simulink model "blinky"  (R2025a)
settings: Solver=FixedStepDiscrete  StartTime=0.0  StopTime=inf  FixedStep=0.001  RelTol=1e-3
model workspace (MAT data in the model file):
  active = Simulink.Parameter
  active.Value = 1
  active.Complexity = 'real'
  active.Dimensions = [1 1]
  active.DataType = 'uint8'
  inactive = Simulink.Parameter
  inactive.Value = 0
  inactive.Complexity = 'real'
  inactive.Dimensions = [1 1]
  inactive.DataType = 'uint8'
undefined symbols (not defined in the file or in its folder): CR, LF, PWM_MAX, PWM_MIN, SPEED_Kd, SPEED_Ki, SPEED_Kp
libraries: instrumentseriallib x3, slpidlib x2, simulink x1, SignalEditorBlockLib x1
settings Model: DataDictionary=control_motor.sldd  Creator=g'w'c  LastModifiedBy=g'w'c
settings OptimizationCC: DefaultParameterBehavior=Inlined  UseDivisionForNetSlopeComputation=on  GainParamInheritBuiltInType=on  UseFloatMulNetSlope=on  DefaultUnderspecifiedDataType=single  InlineInvariantSignals=on  PassReuseOutputArgsAs=Individual arguments  ActiveStateOutputEnumStorageType=uint8  ZeroExternalMemoryAtStartup=off  ZeroInternalMemoryAtStartup=off  NoFixptDivByZeroProtection=on  EfficientFloat2IntCast=on  LifeSpan=1  OptimizeBlockOrder=speed  DifferentSizesBufferReuse=on  EfficientTunableParamExpr=on
settings DebuggingCC: ParameterTunabilityLossMsg=error
settings HardwareCC: ProdLongLongMode=on
settings SFSimCC: MATLABDynamicMemAlloc=off
settings RTWCC: SystemTargetFile=ert.tlc  GenCodeOnly=on  TemplateMakefile=ert_default_tmf  GenerateReport=on  IncludeHyperlinkInReport=on  LaunchReport=on  GenerateTraceInfo=on  GenerateCodeMetricsReport=on  Description=Embedded Coder
settings CodeAppCC: ForceParamTrailComments=on  IgnoreCustomStorageClasses=off  OperatorAnnotations=on  SimulinkDataObjDesc=on  SFDataObjDesc=on  CustomSymbolStrGlobalVar=rt$N$M  CustomSymbolStrType=$N$M  CustomSymbolStrFcn=$N$M$F  CustomSymbolStrMacro=$N$M  InsertBlockDesc=on
settings ERTTargetCC: ExtModeTransport=0.0  ExtModeStaticAlloc=off  ExtModeMexFile=ext_comm  ExtModeIntrfLevel=Level1  ERTCustomFileTemplate=example_file_process.tlc  ERTFilePackagingFormat=CompactWithDataFile  TargetLangStandard=C99 (ISO)  GenerateSampleERTMain=on  IncludeMdlTerminateFcn=off  CombineSignalStateStructs=on  PurelyIntegerCode=on  SupportNonFinite=off  SupportComplex=off  SupportNonInlinedSFcns=on

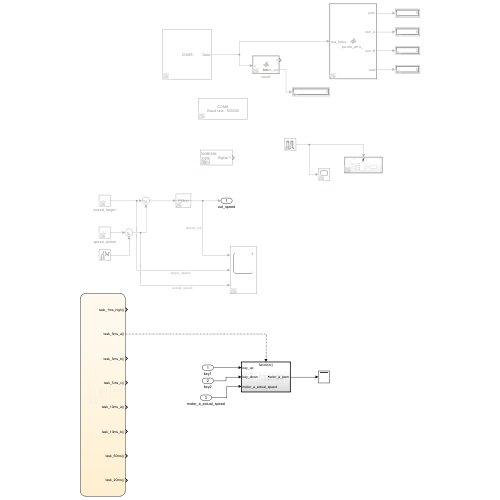
[thumbnail: Simulink's stored preview of the top-level diagram]
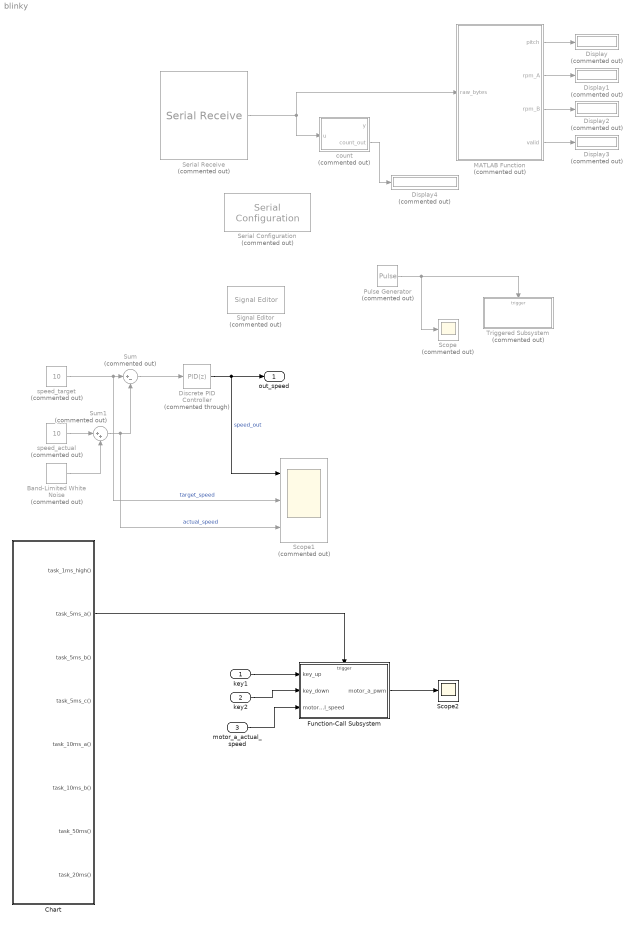
== system blinky ==
  key1 : Inport
  key2 : Inport  Port=2
  motor_a_actual_speed : Inport  Port=3
  Band-Limited White Noise : simulink/Sources/Band-Limited White Noise  Commented=on  Cov=[0.1]  Ts=0.1  seed=[23341]
  Chart : Stateflow chart  TreatAsAtomicUnit=on
  Discrete PID Controller : slpidlib/PID Controller  Commented=through  Controller=PID  Form=Parallel  TimeDomain=Discrete-time  UseExternalTs=off  SampleTime=-1  IntegratorMethod=Forward Euler  FilterMethod=Forward Euler  ControllerParametersSource=internal  P=1  I=1  UseKiTs=off  D=0  UseExternalDerivativeSource=off  N=100  UseFilter=on  TunerSelectOption=Transfer Function Based (PID Tuner App)  InitialConditionSource=internal  InitialConditionForIntegrator=0  InitialConditionForFilter=0  DifferentiatorICPrevScaledInput=0  ExternalReset=none  TrackingMode=off  Kt=1  LimitOutput=off  SatLimitsSource=internal  UpperSaturationLimit=inf  LowerSaturationLimit=-inf  LinearizeAsGain=off  AntiWindupMode=none  Kb=1  LimitIntegrator=off  UpperIntegratorSaturationLimit=inf  LowerIntegratorSaturationLimit=-inf  POutMin=[]  POutMax=[]  IOutMin=[]  IOutMax=[]  DOutMin=[]  DOutMax=[]  NOutMin=[]  NOutMax=[]  SumOutMin=[]  SumOutMax=[]  SaturationOutMin=[]  SaturationOutMax=[]  PParamMin=[]  PParamMax=[]  IParamMin=[]  IParamMax=[]  DParamMin=[]  DParamMax=[]  NParamMin=[]  NParamMax=[]  KbParamMin=[]  KbParamMax=[]  KtParamMin=[]  KtParamMax=[]  KbOutMin=[]  KbOutMax=[]  KtOutMin=[]  KtOutMax=[]  IntegratorOutMin=[]  IntegratorOutMax=[]  FilterOutMin=[]  FilterOutMax=[]  SumI1OutMin=[]  SumI1OutMax=[]  SumI2OutMin=[]  SumI2OutMax=[]  SumI3OutMin=[]  SumI3OutMax=[]  SumI4OutMin=[]  SumI4OutMax=[]  SumDOutMin=[]  SumDOutMax=[]  DifferentiatorOutMin=[]  DifferentiatorOutMax=[]  FilterDiffOutCoefMin=[]  FilterDiffOutCoefMax=[]  ReciprocalOutMin=[]  ReciprocalOutMax=[]  SumDenOutMin=[]  SumDenOutMax=[]  SumNumOutMin=[]  SumNumOutMax=[]  DivideOutMin=[]  DivideOutMax=[]  UdiffTsProdOutMin=[]  UdiffTsProdOutMax=[]  NTsProdOutMin=[]  NTsProdOutMax=[]  UintegralTsProdOutMin=[]  UintegralTsProdOutMax=[]  UngainTsProdOutMin=[]  UngainTsProdOutMax=[]  ClampingZeroOutDataTypeStr=Inherit: Inherit via back propagation  ClampingZeroOutMin=[]  ClampingZeroOutMax=[]  FilterDenConstantOutDataTypeStr=Inherit: Inherit via back propagation  FilterDenConstantOutMin=[]  FilterDenConstantOutMax=[]  PCopyOutDataTypeStr=Inherit: Inherit via back propagation  PCopyOutMin=[]  PCopyOutMax=[]  NCopyOutDataTypeStr=Inherit: Inherit via back propagation  NCopyOutMin=[]  NCopyOutMax=[]  IntegratorContinuousStateAttributes=''  IntegratorStateMustResolveToSignalObject=off  IntegratorRTWStateStorageClass=Auto  FilterContinuousStateAttributes=''  FilterStateMustResolveToSignalObject=off  FilterRTWStateStorageClass=Auto  ParallelPVariant=InternalParameters  IdealPVariant=Disabled  IVariant=InternalParameters  DVariant=InternalParameters  IntegratorVariant=Discrete  SatVariant=Disabled  AWVariant=Passthrough  PCopyVariant=Disabled  TRVariant=Disabled  FdbkBlocksVariant=Forward  IdealPFdbkVariant=Disabled  SatFdbkVariant=Disabled  DerivativeFilterVariant=ForwardEulerFilter  NVariant=InternalParameters  NCopyVariant=Disabled  FilterICVariant=InternalICsFilter  IntegratorICVariant=InternalICs  ExternalResetVariant=Disabled  TRSumVariant=Passthrough  SumFdbkVariant=Disabled  SumVariant=Sum_PID  TsampFilterVariant=InternalTs  TsampNgainVariant=Passthrough  TsampIntegralVariant=Disabled_SignalSpec  ExternalSaturationOutDataTypeStr=Inherit: Same as second input  DerivativeSourceVariant=ErrorSignal  PreIntVariant=InternalPreInt
      settings: LibrarySourceBlock=simulink/Discrete/Discrete PID Controller
  Display{,1..4} (5 alike) : Display  Commented=on
      Display4 settings: Format=decimal (Stored Integer)
  Function-Call Subsystem : Subsystem  TreatAsAtomicUnit=on
  MATLAB Function : MATLAB Function  Commented=on  TreatAsAtomicUnit=on
  Pulse Generator : DiscretePulseGenerator  Commented=on  PulseType=Time based  Period=1
  Scope : Scope  Commented=on
      settings: ActiveDisplayYMinimum=-4.2942185236028347  ActiveDisplayYMaximum=2.5004399483972364
  Scope1 : Scope  Commented=on  NumInputPorts=3
      settings: ActiveDisplayYMinimum=-1.2558823787460671E+274  ActiveDisplayYMaximum=2.7568149777352689E+273
  Scope2 : Scope
      settings: DataLoggingVariableName=ScopeData3
  Serial Configuration : instrumentseriallib/Serial Configuration  Priority=-200000  Commented=on  PortSel=COM8  Port=COM8  ComPort=COM8  BaudRate=500000  DataBits=8  Parity=none  StopBits=1  ByteOrder=little-endian  FlowControl=none  Timeout=10  SimulateUsing=Interpreted execution  BlockInModel=on  aMode=1
  Serial Receive : instrumentseriallib/Serial Receive  Priority=1  Commented=on  PortSel=COM8  Port=COM8  ComPort=COM8  DataType=uint8  SaveDataType=uint8  ToggleHeader=on  Header=[170 255]  ToggleDataSize=on  DataSize=[1 30]  ToggleTerminator=off  Terminator=CR/LF ('\r\n')  CustomTerminator=[]  InputFormat=Column major  EnableBlockingMode=on  ActionDataUnavailable=Output last received value  ActionWhenDataUnavailable=Output last received value  CustomValue=0  SampleTime=0.01  SimulateUsing=Interpreted execution  BlockInModel=on  aMode=1  LibraryInUse=instrumentlib
  Signal Editor : SignalEditorBlockLib/Signal Editor  Commented=on  FileName=com_uart.mat  ActiveScenario=Scenario  ActiveSignal=Signal 1  IsBus=off  OutputBusObjectStr=Bus: BusObject  SampleTime=0  ZeroCross=off  OutputAfterFinalValue=Setting to zero  Unit=inherit  PreserveSignalName=on  ApplySigPropsToAllScenarios=on  ApplySigPropsToAllSignals=off  SignalPropertySource=Dialog parameters
  Sum : Sum  Commented=on  Inputs=|+-
  Sum1 : Sum  Commented=on  Inputs=|++
  Triggered Subsystem : Subsystem  Commented=on  TreatAsAtomicUnit=on
  count : MATLAB Function  Commented=on  TreatAsAtomicUnit=on
  speed_actual : Constant  Commented=on  Value=10
  speed_target : Constant  Commented=on  Value=10
  out_speed : Outport
  wires:
  Serial Receive/1 -> MATLAB Function/1(raw_bytes), count/1(u)
  Pulse Generator/1 -> Triggered Subsystem/Trigger, Scope/1
  count/2(count_out) -> Display4/1
  MATLAB Function/1(pitch) -> Display/1
  MATLAB Function/2(rpm_A) -> Display1/1
  MATLAB Function/3(rpm_B) -> Display2/1
  MATLAB Function/4(valid) -> Display3/1
  speed_target/1 -> Scope1/2, Sum/1  "target_speed"
  Sum/1 -> Discrete PID Controller/1
  speed_actual/1 -> Sum1/1
  Band-Limited White Noise/1 -> Sum1/2
  Sum1/1 -> Scope1/3, Sum/2  "actual_speed"
  Discrete PID Controller/1 -> Scope1/1, out_speed/1  "speed_out"
  Chart/2(task_5ms_a()) -> Function-Call Subsystem/Trigger
  key1/1 -> Function-Call Subsystem/1(key_up)
  key2/1 -> Function-Call Subsystem/2(key_down)
  motor_a_actual_speed/1 -> Function-Call Subsystem/3(motor_a_actual_speed)
  Function-Call Subsystem/1(motor_a_pwm) -> Scope2/1

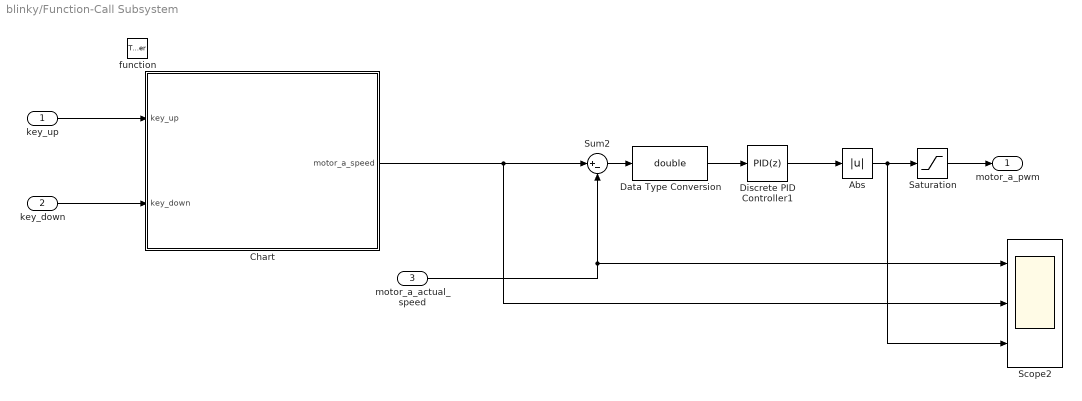
== system blinky/Function-Call Subsystem ==
  key_up : Inport
  key_down : Inport  Port=2
  motor_a_actual_speed : Inport  Port=3
  function : TriggerPort  TriggerType=function-call  VariantControl=(inherit)
  Abs : Abs  SaturateOnIntegerOverflow=off
  Chart : Stateflow chart  TreatAsAtomicUnit=on
  Data Type Conversion : DataTypeConversion  OutDataTypeStr=double  SaturateOnIntegerOverflow=off  RndMeth=Floor
  Discrete PID Controller1 : slpidlib/PID Controller  Controller=PID  Form=Parallel  TimeDomain=Discrete-time  UseExternalTs=off  SampleTime=-1  IntegratorMethod=Forward Euler  FilterMethod=Forward Euler  ControllerParametersSource=internal  P=SPEED_Kp  I=SPEED_Ki  UseKiTs=off  D=SPEED_Kd  UseExternalDerivativeSource=off  N=100  UseFilter=on  TunerSelectOption=Transfer Function Based (PID Tuner App)  InitialConditionSource=internal  InitialConditionForIntegrator=0  InitialConditionForFilter=0  DifferentiatorICPrevScaledInput=0  ExternalReset=none  TrackingMode=off  Kt=1  LimitOutput=off  SatLimitsSource=internal  UpperSaturationLimit=inf  LowerSaturationLimit=-inf  LinearizeAsGain=off  AntiWindupMode=none  Kb=1  LimitIntegrator=off  UpperIntegratorSaturationLimit=inf  LowerIntegratorSaturationLimit=-inf  POutMin=[]  POutMax=[]  IOutMin=[]  IOutMax=[]  DOutMin=[]  DOutMax=[]  NOutMin=[]  NOutMax=[]  SumOutMin=[]  SumOutMax=[]  SaturationOutMin=[]  SaturationOutMax=[]  PParamMin=[]  PParamMax=[]  IParamMin=[]  IParamMax=[]  DParamMin=[]  DParamMax=[]  NParamMin=[]  NParamMax=[]  KbParamMin=[]  KbParamMax=[]  KtParamMin=[]  KtParamMax=[]  KbOutMin=[]  KbOutMax=[]  KtOutMin=[]  KtOutMax=[]  IntegratorOutMin=[]  IntegratorOutMax=[]  FilterOutMin=[]  FilterOutMax=[]  SumI1OutMin=[]  SumI1OutMax=[]  SumI2OutMin=[]  SumI2OutMax=[]  SumI3OutMin=[]  SumI3OutMax=[]  SumI4OutMin=[]  SumI4OutMax=[]  SumDOutMin=[]  SumDOutMax=[]  DifferentiatorOutMin=[]  DifferentiatorOutMax=[]  FilterDiffOutCoefMin=[]  FilterDiffOutCoefMax=[]  ReciprocalOutMin=[]  ReciprocalOutMax=[]  SumDenOutMin=[]  SumDenOutMax=[]  SumNumOutMin=[]  SumNumOutMax=[]  DivideOutMin=[]  DivideOutMax=[]  UdiffTsProdOutMin=[]  UdiffTsProdOutMax=[]  NTsProdOutMin=[]  NTsProdOutMax=[]  UintegralTsProdOutMin=[]  UintegralTsProdOutMax=[]  UngainTsProdOutMin=[]  UngainTsProdOutMax=[]  ClampingZeroOutDataTypeStr=Inherit: Inherit via back propagation  ClampingZeroOutMin=[]  ClampingZeroOutMax=[]  FilterDenConstantOutDataTypeStr=Inherit: Inherit via back propagation  FilterDenConstantOutMin=[]  FilterDenConstantOutMax=[]  PCopyOutDataTypeStr=Inherit: Inherit via back propagation  PCopyOutMin=[]  PCopyOutMax=[]  NCopyOutDataTypeStr=Inherit: Inherit via back propagation  NCopyOutMin=[]  NCopyOutMax=[]  IntegratorContinuousStateAttributes=''  IntegratorStateMustResolveToSignalObject=off  IntegratorRTWStateStorageClass=Auto  FilterContinuousStateAttributes=''  FilterStateMustResolveToSignalObject=off  FilterRTWStateStorageClass=Auto  ParallelPVariant=InternalParameters  IdealPVariant=Disabled  IVariant=InternalParameters  DVariant=InternalParameters  IntegratorVariant=Discrete  SatVariant=Disabled  AWVariant=Passthrough  PCopyVariant=Disabled  TRVariant=Disabled  FdbkBlocksVariant=Forward  IdealPFdbkVariant=Disabled  SatFdbkVariant=Disabled  DerivativeFilterVariant=ForwardEulerFilter  NVariant=InternalParameters  NCopyVariant=Disabled  FilterICVariant=InternalICsFilter  IntegratorICVariant=InternalICs  ExternalResetVariant=Disabled  TRSumVariant=Passthrough  SumFdbkVariant=Disabled  SumVariant=Sum_PID  TsampFilterVariant=InternalTs  TsampNgainVariant=Passthrough  TsampIntegralVariant=Disabled_SignalSpec  ExternalSaturationOutDataTypeStr=Inherit: Same as second input  DerivativeSourceVariant=ErrorSignal  PreIntVariant=InternalPreInt
      settings: LibrarySourceBlock=simulink/Discrete/Discrete PID Controller
  Saturation : Saturate  UpperLimit=PWM_MAX  LowerLimit=PWM_MIN
  Scope2 : Scope  NumInputPorts=3
      settings: DataLoggingVariableName=ScopeData2
  Sum2 : Sum  Inputs=|+-
  motor_a_pwm : Outport
  wires:
  key_up/1 -> Chart/1(key_up)
  key_down/1 -> Chart/2(key_down)
  Sum2/1 -> Data Type Conversion/1
  Chart/1(motor_a_speed) -> Sum2/1, Scope2/2
  Saturation/1 -> motor_a_pwm/1
  Data Type Conversion/1 -> Discrete PID Controller1/1
  Abs/1 -> Scope2/3, Saturation/1
  Discrete PID Controller1/1 -> Abs/1
  motor_a_actual_speed/1 -> Scope2/1, Sum2/2

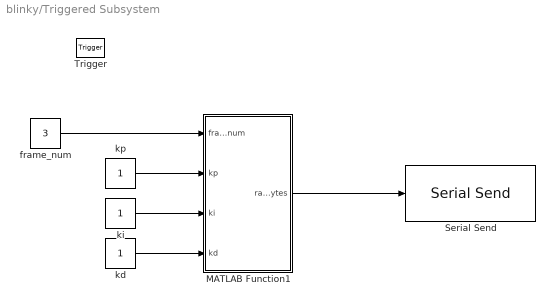
== system blinky/Triggered Subsystem ==
  Trigger : TriggerPort  VariantControl=(inherit)
  MATLAB Function1 : MATLAB Function  TreatAsAtomicUnit=on
  Serial Send : instrumentseriallib/Serial Send  Priority=1  PortSel=COM8  Port=COM8  ComPort=COM8  Header=[]  Terminator=<none>  CustomTerminator=[]  EnableBlockingMode=off  SimulateUsing=Interpreted execution  BlockInModel=on  aMode=1
      settings: LibrarySourceBlock=c2000lib/Host Communication/Serial Send
  frame_num : Constant  Value=3  OutDataTypeStr=uint8
  kd : Constant  OutDataTypeStr=single
  ki : Constant  OutDataTypeStr=single
  kp : Constant  OutDataTypeStr=single
  wires:
  kp/1 -> MATLAB Function1/2(kp)
  frame_num/1 -> MATLAB Function1/1(frame_num)
  ki/1 -> MATLAB Function1/3(ki)
  kd/1 -> MATLAB Function1/4(kd)
  MATLAB Function1/1(raw_bytes) -> Serial Send/1

== matlab function blinky/Triggered Subsystem/MATLAB Function1 ==
  data: frame_num input; raw_bytes output; kp input; ki input; kd input
function raw_bytes = ano_send(frame_num, kp, ki, kd)

    FRAME_HEADER = 0xAA;
    TARGET_ADDR  = 0xFF;
    SCALE_FACTOR = 1000;
    
    kp_int = int32(round(kp * SCALE_FACTOR));
    ki_int = int32(round(ki * SCALE_FACTOR));
    kd_int = int32(round(kd * SCALE_FACTOR));
    
    tx_buffer = uint8(zeros(1, 64));
    cnt = 1;
    
    tx_buffer(cnt) = FRAME_HEADER; cnt = cnt + 1;
    tx_buffer(cnt) = TARGET_ADDR; cnt = cnt + 1;
    tx_buffer(cnt) = uint8(frame_num); cnt = cnt + 1;
    
    len_idx = cnt;
    tx_buffer(cnt) = 0; cnt = cnt + 1;
    
    tx_buffer(cnt:cnt+3) = int32_to_bytes_le(kp_int); cnt = cnt + 4;
    tx_buffer(cnt:cnt+3) = int32_to_bytes_le(ki_int); cnt = cnt + 4;
    tx_buffer(cnt:cnt+3) = int32_to_bytes_le(kd_int); cnt = cnt + 4;
    
    data_len = cnt - 5;
    tx_buffer(len_idx) = uint8(data_len);
    
    % ========== 校验计算（修复溢出警告）==========
    check_sum1 = uint16(0);   % 用 uint16 累加
    check_sum2 = uint16(0);
    
    for i = 1:(cnt - 1)
        check_sum1 = check_sum1 + uint16(tx_buffer(i));
        check_sum2 = check_sum2 + check_sum1;
    end
    
    % 截断为 8 位，模拟 C 的溢出回绕
    tx_buffer(cnt) = uint8(bitand(check_sum1, uint16(0xFF))); cnt = cnt + 1;
    tx_buffer(cnt) = uint8(bitand(check_sum2, uint16(0xFF))); cnt = cnt + 1;
    
    raw_bytes = tx_buffer(1:(cnt - 1));
end

function bytes = int32_to_bytes_le(val)
    bytes = uint8(zeros(1, 4));
    bytes(1) = uint8(bitand(val, int32(0x000000FF)));
    bytes(2) = uint8(bitand(bitshift(val, -8), int32(0xFF)));
    bytes(3) = uint8(bitand(bitshift(val, -16), int32(0xFF)));
    bytes(4) = uint8(bitand(bitshift(val, -24), int32(0xFF)));
end

== matlab function blinky/MATLAB Function ==
  data: raw_bytes input; pitch output; rpm_A output; rpm_B output; valid output
function [pitch, rpm_A, rpm_B, valid] = parse_ano_(raw_bytes)  
    % 输出初始化
    pitch = 0.0;
    rpm_A = single(0);
    rpm_B = single(0);
    valid = false;

    % pitch (double, 8字节)
    p_bytes = zeros(1, 8, 'uint8');

    for i = uint8(1):uint8(8)
        p_bytes(i) = raw_bytes(i + uint8(2));
    end
    pitch = typecast(p_bytes, 'double');

    % rpm_A (float, 4字节)
    ra_bytes = zeros(1, 4, 'uint8');
    for i = uint8(1):uint8(4)
        ra_bytes(i) = raw_bytes(uint8(8) + i + uint8(2));
    end
    rpm_A = typecast(ra_bytes, 'single');

    % rpm_B (float, 4字节)
    rb_bytes = zeros(1, 4, 'uint8');
    for i = uint8(1):uint8(4)
        rb_bytes(i) = raw_bytes(uint8(12) + i + uint8(2));
    end
    rpm_B = typecast(rb_bytes, 'single');

    

        % 校验失败或不是目标帧，继续
end

== matlab function blinky/count ==
  data: u input; y output; count_out output
function [y, count_out] = fcn(u)
    persistent n;
    if isempty(n)
        n = 0;
    end
    n = n + 1;
    count_out = double(n);  % 确保类型是 double
    y = u;
end

== stateflow chart blinky/Chart ==
  note: 整个chart只是为了释放事件而使用
  state task_10ms_high [function]
    (default) -> (junction 107)
    (junction 107) -> (junction 110) [order 1] : [task_10ms_count == 1]
    (junction 107) -> (junction 118) [order 2]
    (junction 110) -> (junction 117) : {task_10ms_a}
    (junction 117) -> (junction 118)
    (junction 118) -> (junction 120)
    (junction 120) -> (junction 113) [order 1] : [task_10ms_count == 2]
    (junction 120) -> (junction 115) [order 2]
    (junction 113) -> (junction 105) : {task_10ms_b}
    (junction 105) -> (junction 115)
  state task_5ms_high [function]
    (default) -> (junction 50)
    (junction 50) -> (junction 52) [order 1] : [task_5ms_count == 1]
    (junction 50) -> (junction 54) [order 2]
    (junction 52) -> (junction 56) : {task_5ms_a}
    (junction 56) -> (junction 54)
    (junction 54) -> (junction 59)
    (junction 59) -> (junction 61) [order 1] : [task_5ms_count == 2]
    (junction 59) -> (junction 63) [order 2]
    (junction 61) -> (junction 64) : {task_5ms_b}
    (junction 64) -> (junction 63)
    (junction 63) -> (junction 68)
    (junction 68) -> (junction 71) [order 1] : [task_5ms_count == 3]
    (junction 68) -> (junction 75) [order 2]
    (junction 71) -> (junction 73) : {task_5ms_c}
    (junction 73) -> (junction 75)
  state task_20ms_high [function]
    (default) -> (junction 130)
    (junction 130) -> (junction 129) [order 1] : [task_20ms_count == 1]
    (junction 130) -> (junction 131) [order 2]
    (junction 129) -> (junction 122) : {task_20ms}
    (junction 122) -> (junction 131)
  state task_50ms_high [function]
    (default) -> (junction 139)
    (junction 139) -> (junction 125) [order 1] : [task_50ms_count == 1]
    (junction 139) -> (junction 126) [order 2]
    (junction 125) -> (junction 123) : {task_50ms}
    (junction 123) -> (junction 126)
  note: 创建任务的状态机系统罢了
  (default) -> (junction 1) : {task_5ms_count = task_5ms_count + 1;}
  (junction 1) -> (junction 5) : {task_1ms_high}
  (junction 5) -> (junction 6) [order 1] : [mod(task_5ms_count,5) == 0]
  (junction 5) -> (junction 10) [order 2]
  (junction 6) -> (junction 8) : {task_5ms_count = 0;}
  (junction 8) -> (junction 10)
  (junction 10) -> (junction 14) : {task_10ms_count = task_10ms_count + 1;}
  (junction 14) -> (junction 16) [order 1] : [mod(task_10ms_count,10)==0]
  (junction 14) -> (junction 20) [order 2]
  (junction 16) -> (junction 18) : {task_10ms_count = 0;}
  (junction 18) -> (junction 20)
  (junction 20) -> (junction 23) : {task_20ms_count = task_20ms_count + 1;}
  (junction 23) -> (junction 25) [order 1] : [mod(task_20ms_count,20) == 0]
  (junction 23) -> (junction 29) [order 2]
  (junction 25) -> (junction 27) : {task_20ms_count = 0;}
  (junction 27) -> (junction 29)
  (junction 29) -> (junction 33) : {task_50ms_count = task_50ms_count + 1;}
  (junction 33) -> (junction 35) [order 1] : [mod(task_50ms_count,50) == 0]
  (junction 33) -> (junction 39) [order 2]
  (junction 35) -> (junction 37) : {task_50ms_count = 0;}
  (junction 37) -> (junction 39)
  (junction 39) -> (junction 42) : {task_5ms_high();
      | task_10ms_high();
      | task_20ms_high();
      | task_50ms_high();
      | }
  data: task_10ms_count local =0; task_5ms_count local =0; task_50ms_count local =0; task_20ms_count local =0
  events: task_1ms_high output FUNCTION_CALL_EVENT; task_5ms_a output FUNCTION_CALL_EVENT; task_5ms_b output FUNCTION_CALL_EVENT; task_5ms_c output FUNCTION_CALL_EVENT; task_10ms_a output FUNCTION_CALL_EVENT; task_10ms_b output FUNCTION_CALL_EVENT; task_50ms output FUNCTION_CALL_EVENT; task_20ms output FUNCTION_CALL_EVENT

== stateflow chart blinky/Function-Call Subsystem/Chart ==
  state speed_down [function]
    (default) -> (junction 22)
    (junction 22) -> (junction 16) [order 1] : [key_down == ON]
    (junction 22) -> (junction 25) [order 2]
    (junction 16) -> (junction 17) : {motor_a_speed = motor_a_speed - 20;}
    (junction 25) -> (junction 17)
  state speed_up [function]
    (default) -> (junction 2)
    (junction 2) -> (junction 7) [order 1] : [key_up == ON]
    (junction 2) -> (junction 12) [order 2]
    (junction 7) -> (junction 10) : {motor_a_speed = motor_a_speed + 20;}
    (junction 12) -> (junction 10)
  state speed_staus
    en:
    motor_a_speed = 0;
    du:
    speed_up();
    speed_down();
  (default) -> speed_staus
  data: key_up input uint8; key_down input uint8; ON parameter uint8 size=1; motor_a_speed output
